simulink model "verify_clq2friction_coeff_mdl"  (R2018b)
settings: Solver=VariableStepDiscrete  StartTime=0.0  StopTime=10.0  MaxStep=0.1  RelTol=1e-3  EnableMultiTasking=on
libraries: carnot x4, simulink x1
settings Model: Creator=drhf  LastModifiedBy=drhf
settings DataIOCC: LimitDataPoints=on  SaveFormat=Array
settings OptimizationCC: ExpressionDepthLimit=2147483647  LifeSpan=inf
settings DebuggingCC: UnderspecifiedInitializationDetection=Classic  MergeDetectMultiDrivingBlocksExec=none  SolverPrmCheckMsg=warning  StateNameClashWarn=warning  SFUnexpectedBacktrackingDiag=warning  SFNoUnconditionalDefaultTransitionDiag=warning  SFExecutionAtInitializationDiag=none
settings HardwareCC: ProdBitPerPointer=32  ProdBitPerSizeT=32  ProdBitPerPtrDiffT=32  ProdLargestAtomicFloat=None  ProdIntDivRoundTo=Undefined  ProdEndianess=Unspecified  ProdWordSize=32  ProdHWDeviceType=32-bit Generic
settings ModelReferenceCC: PropagateSignalLabelsOutOfModel=off
settings SFSimCC: SimUseLocalCustomCode=off
settings RTWCC: RTWUseLocalCustomCode=off
settings CodeAppCC: StateflowObjectComments=on
settings GRTTargetCC: TargetLangStandard=C89/C90 (ANSI)  GeneratePreprocessorConditionals=Disable all  CombineOutputUpdateFcns=off  GRTInterface=on
settings ConfigComp: CovMetricSettings=dw  CovHtmlReporting=on  CovSaveCumulativeToWorkspaceVar=on  CovSaveSingleToWorkspaceVar=on  CovExternalEMLEnable=off

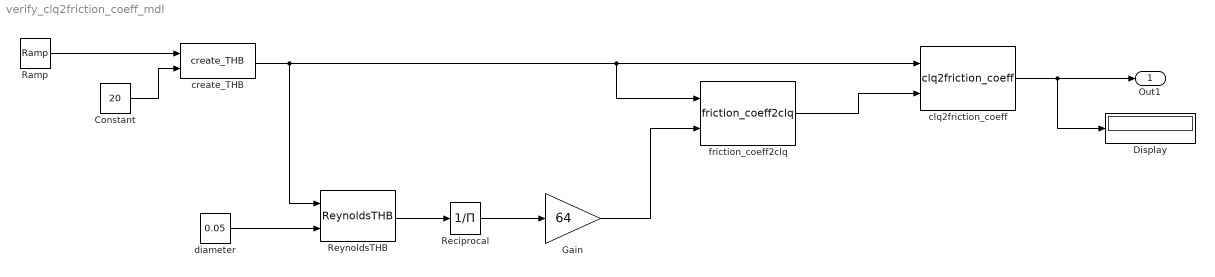
== system verify_clq2friction_coeff_mdl ==
  Constant : Constant  Value=20
  Display : Display
  Gain : Gain  Gain=64
  Ramp : simulink/Sources/Ramp  slope=0.01  start=0  InitialOutput=0
  Reciprocal : Product  Inputs=/  SaturateOnIntegerOverflow=on  RndMeth=Zero
  ReynoldsTHB : carnot/Basic/Hydraulics/ReynoldsTHB
      settings: SourceProductName=Carnot
  clq2friction_coeff : carnot/Basic/Pressure_Drop/clq2friction_coeff  Value=0.05  Gain=1
      settings: SourceProductName=Carnot
  create_THB : carnot/Source/Simple/create_THB  p=1e5  fluid=Water  mix=0  mix2=0  mix3=0  dia=0.02  hgt=0  mID=Pressure Drop from Massflow
      settings: SourceProductName=Carnot
  diameter : Constant  Value=0.05
  friction_coeff2clq : carnot/Basic/Pressure_Drop/friction_coeff2clq  Value=0.05  Gain=1
      settings: SourceProductName=Carnot
  Out1 : Outport  SampleTime=1
  wires:
  clq2friction_coeff/1 -> Display/1, Out1/1
  Ramp/1 -> create_THB/1
  Constant/1 -> create_THB/2
  create_THB/1 -> ReynoldsTHB/1, clq2friction_coeff/1, friction_coeff2clq/1
  diameter/1 -> ReynoldsTHB/2
  ReynoldsTHB/1 -> Reciprocal/1
  Reciprocal/1 -> Gain/1
  Gain/1 -> friction_coeff2clq/2
  friction_coeff2clq/1 -> clq2friction_coeff/2
